simulink model "asynchronous_motor_simulation"  (R2017b)
settings: Solver=FixedStepAuto  StartTime=0.0  StopTime=1  FixedStep=0.0001  MaxStep=1e-4  RelTol=1e-3
libraries: powerlib x6
settings Model: Creator=Damla  LastModifiedBy=dagac

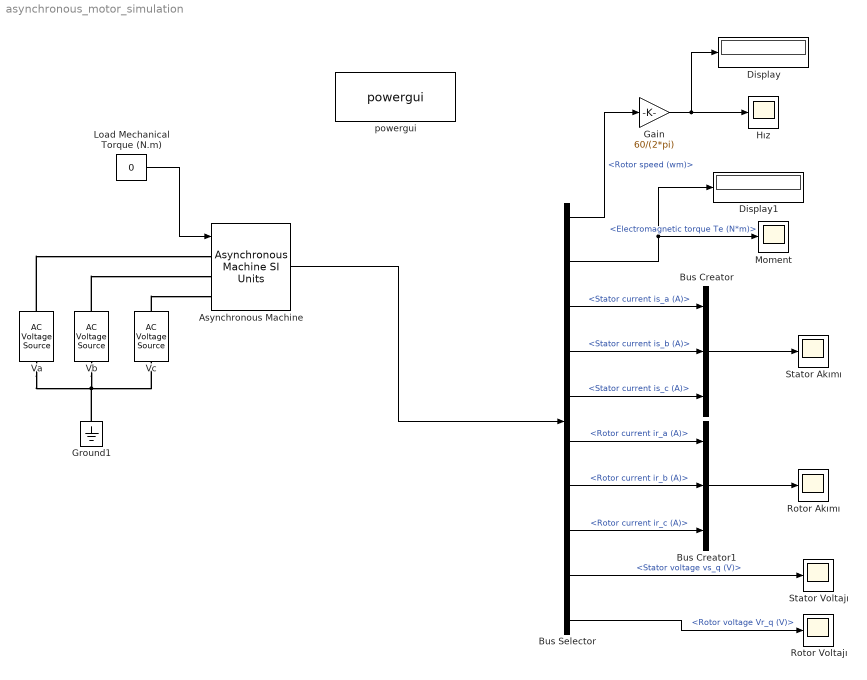
== system asynchronous_motor_simulation ==
  "Asynchronous Machine " : powerlib/Machines/Asynchronous Machine SI Units  RotorType=Squirrel-cage  PresetModel=No  MechanicalLoad=Torque Tm  ShowDetailedParameters=on  ReferenceFrame=Stationary  Units=SI  MeasurementBus=off  NominalParameters=[1100 380 50]  Stator=[9.63 0.02]  Rotor=[5.459 0.03]  Cage1=[ 0.022 0.226/377]  Cage2=[ 0.022 0.226/377]  Lm=0.434  Mechanical=[0.033 0.00413403 2]  PolePairs=2  InitialConditions="[ 1,0   0,0,0   0,0,0 ]"  SimulateSaturation=off  Saturation=[9.9249,19.6672,38.0377,51.3988,69.2824,105.1337,152.5532,214.2421,302;230, 322, 414, 460, 506, 552, 598, 644, 690]  LoadFlowParameters=0  TsPowergui=0  TsBlock=-1  IterativeModel=Trapezoidal non iterative  IterativeDiscreteModel=Trapezoidal non iterative  Pmec=0
  Bus Creator : BusCreator  Inputs=3
  Bus Creator1 : BusCreator  Inputs=3
  Bus Selector : BusSelector  OutputSignals=Mechanical.Rotor speed (wm),Mechanical.Electromagnetic torque Te (N*m),Stator measurements.Stator current is_a (A),Stator measurements.Stator current is_b (A),Stator measurements.Stator current is_c (A),Rotor measurements.Rotor current ir_a (A),Rotor measurements.Rotor current ir_b (A),Rotor measurements.Rotor current ir_c (A),Stator measurements.Stator voltage vs_q (V),Rotor measurements.Rotor voltage Vr_q (V)
  Display : Display
  Display1 : Display
  Gain : Gain  Gain=60/(2*pi)
  Ground1 : powerlib/Elements/Ground  LConnTagsString=a
  Hız : Scope
  Load Mechanical Torque (N.m) : Constant  Value=0
  Moment : Scope
  Rotor Akımı : Scope
  Rotor Voltajı : Scope
  Stator Akımı : Scope
  Stator Voltajı : Scope
  Va : powerlib/Electrical Sources/AC Voltage Source  Amplitude=310.268  Phase=0  Frequency=50  SampleTime=0  Measurements=None  BusType=swing  Pref=10e3  Qref=0  Qmin=-inf  Qmax=+inf
  Vb : powerlib/Electrical Sources/AC Voltage Source  Amplitude=310.268  Phase=-120  Frequency=50  SampleTime=0  Measurements=None  BusType=swing  Pref=10e3  Qref=0  Qmin=-inf  Qmax=+inf
  Vc : powerlib/Electrical Sources/AC Voltage Source  Amplitude=310.268  Phase=120  Frequency=50  SampleTime=0  Measurements=None  BusType=swing  Pref=10e3  Qref=0  Qmin=-inf  Qmax=+inf
  powergui : powerlib/powergui  Priority=1  SimulationMode=Discrete  SampleTime=0.0001  frequency=60  Iterations=50  frequencyindice=50  Pbase=100e6  ErrMax=1e-4  UnitsV=kV  UnitsW=MW  buscounter=0  FunctionMessages=off  echomessages=off  EnableUseOfTLC=off  CurrentSourceSwitches=off  DisableSnubberDevices=off  DisableRonSwitches=off  DisableVfSwitches=off  DisplayEquations=off  SolverType=Tustin/Backward Euler (TBE)  Interpol=off  ExternalGateDelay=off  methode=off  Ts=100  x0status=blocks  SPID=off  SwTol=0  HookPort=off  RestoreLinks=warning  ResistiveCurrentMeasurement=off  Frange=[0:2:500]  Ylog=off  Xlog=on  ShowGrid=off  save=off  variable=ZData  structure=0  ZoomFFT=off  StartTime=0.0  cycles=1  DisplayStyle=1  fundamental=60  FreqAxis=off  MaxFrequency=1000  frequencyindicesteady=1  RmsSteady=1  display=off
  wires:
  Gain/1 -> Display/1, Hız/1
  Bus Selector/10 -> Rotor Voltajı/1  "<Rotor voltage Vr_q (V)>"
  "Asynchronous Machine "/1 -> Bus Selector/1
  Bus Creator/1 -> Stator Akımı/1
  Bus Selector/6 -> Bus Creator1/1  "<Rotor current ir_a (A)>"
  Bus Selector/2 -> Moment/1, Display1/1  "<Electromagnetic torque Te (N*m)>"
  Bus Selector/9 -> Stator Voltajı/1  "<Stator voltage vs_q (V)>"
  Bus Selector/8 -> Bus Creator1/3  "<Rotor current ir_c (A)>"
  Bus Creator1/1 -> Rotor Akımı/1
  Bus Selector/7 -> Bus Creator1/2  "<Rotor current ir_b (A)>"
  Bus Selector/4 -> Bus Creator/2  "<Stator current is_b (A)>"
  Bus Selector/1 -> Gain/1  "<Rotor speed (wm)>"
  Bus Selector/3 -> Bus Creator/1  "<Stator current is_a (A)>"
  Load Mechanical Torque (N.m)/1 -> "Asynchronous Machine "/1
  Bus Selector/5 -> Bus Creator/3  "<Stator current is_c (A)>"
  connections:
  Ground1/LConn1 -- Va/LConn1 -- Vc/LConn1 -- Vb/LConn1
  Vc/RConn1 -- "Asynchronous Machine "/LConn3
  Va/RConn1 -- "Asynchronous Machine "/LConn1
  Vb/RConn1 -- "Asynchronous Machine "/LConn2
